simulink model "detailed"  (Simulink 8.1)
settings: Solver=ode4  StartTime=0.0  StopTime=inf  FixedStep=0.01  RelTol=1e-3
values from neighbouring files (symbols this model uses):
  fc = 1    [parametry.m]
  fp = 0.5    [parametry.m]
  g = 9.81    [parametry.m]
  l = 0.165    [parametry.m]
  m = 0.192    [parametry.m]
  M = 0.604    [parametry.m]
  theta0 = 0    [suwnica.m]
  thetaprim0 = 0.05    [suwnica.m]
  x0 = [x0 xprim0 theta0 thetaprim0]    [suwnica.m]
  xprim0 = 0    [suwnica.m]
libraries: simulink x1
settings Model: Creator=Michał  LastModifiedBy=Michał  SimulationMode=rapid-accelerator
settings DataIOCC: SignalLoggingSaveFormat=Dataset
settings OptimizationCC: ExpressionDepthLimit=128
settings DebuggingCC: FcnCallInpInsideContextMsg=EnableAllAsError
settings GRTTargetCC: CombineOutputUpdateFcns=on  GRTInterface=off

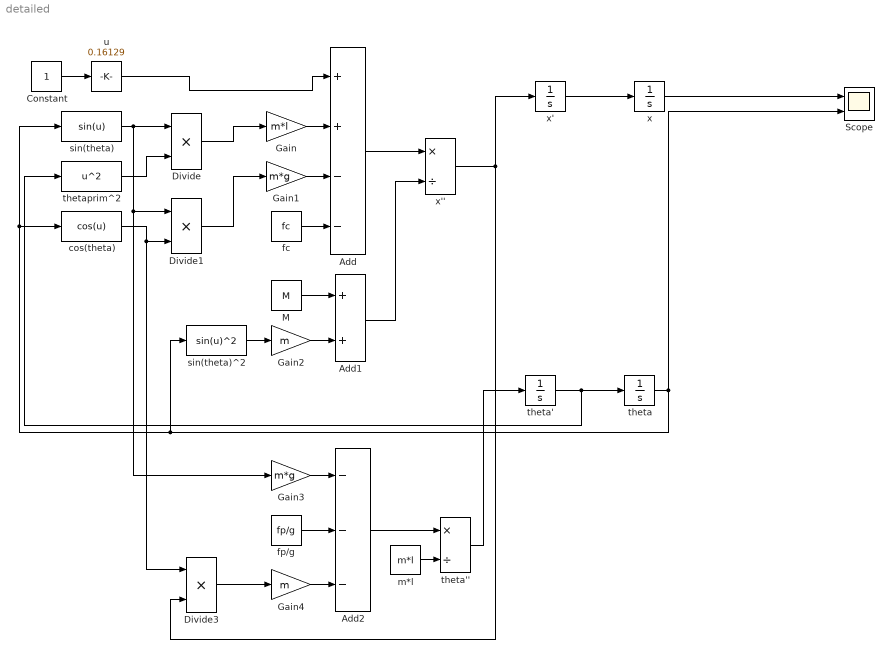
== system detailed ==
  Add : Sum  Inputs=++--
  Add1 : Sum
  Add2 : Sum  Inputs=---
  Constant : Constant
  Divide : Product  Inputs=**
  Divide1 : Product  Inputs=**
  Divide3 : Product  Inputs=**
  Gain : Gain  Gain=m*l
  Gain1 : Gain  Gain=m*g
  Gain2 : Gain  Gain=m
  Gain3 : Gain  Gain=m*g
  Gain4 : Gain  Gain=m
  M : Constant  Value=M
  Scope : Scope  NumInputPorts=2
      settings: YMin=-1.562e+07~-5  YMax=-1.55e+07~5
  "cos(theta) " : Fcn  Expr=cos(u)
  fc : Constant  Value=fc
  fp/g : Constant  Value=fp/g
  m*l : Constant  Value=m*l
  sin(theta) : Fcn  Expr=sin(u)
  sin(theta)^2 : Fcn  Expr=sin(u)^2
  theta : Integrator  InitialCondition=theta0
  theta' : Integrator  InitialCondition=thetaprim0
  theta'' : Product  Inputs=*/
  thetaprim^2 : Fcn  Expr=u^2
  u : simulink/Math Operations/Slider Gain  low=-5  gain=0.16129  high=5
  x : Integrator  InitialCondition=x0
  x' : Integrator  InitialCondition=xprim0
  x'' : Product  Inputs=*/
  wires:
  x'/1 -> x/1
  theta'/1 -> thetaprim^2/1, theta/1
  Constant/1 -> u/1
  Gain/1 -> Add/2
  Divide/1 -> Gain/1
  thetaprim^2/1 -> Divide/2
  sin(theta)/1 -> Gain3/1, Divide1/1, Divide/1
  Gain1/1 -> Add/3
  Divide1/1 -> Gain1/1
  "cos(theta) "/1 -> Divide3/1, Divide1/2
  fc/1 -> Add/4
  M/1 -> Add1/1
  Gain2/1 -> Add1/2
  sin(theta)^2/1 -> Gain2/1
  Add/1 -> x''/1
  Add1/1 -> x''/2
  x''/1 -> Divide3/2, x'/1
  x/1 -> Scope/1
  theta/1 -> sin(theta)^2/1, "cos(theta) "/1, sin(theta)/1, Scope/2
  Gain3/1 -> Add2/1
  fp/g/1 -> Add2/2
  Gain4/1 -> Add2/3
  Divide3/1 -> Gain4/1
  Add2/1 -> theta''/1
  theta''/1 -> theta'/1
  m*l/1 -> theta''/2
  u/1 -> Add/1
